simulink model "Verification_Controller_Tank2_Primitive"  (R2012b)
settings: Solver=FixedStepDiscrete  StartTime=0.0  StopTime=10.0  FixedStep=0.1  RelTol=1e-3
libraries: sldvlib x15
settings Model: Creator=Kerianne  LastModifiedBy=Kerianne
settings DataIOCC: SaveFormat=Structure
settings OptimizationCC: InlineParams=on

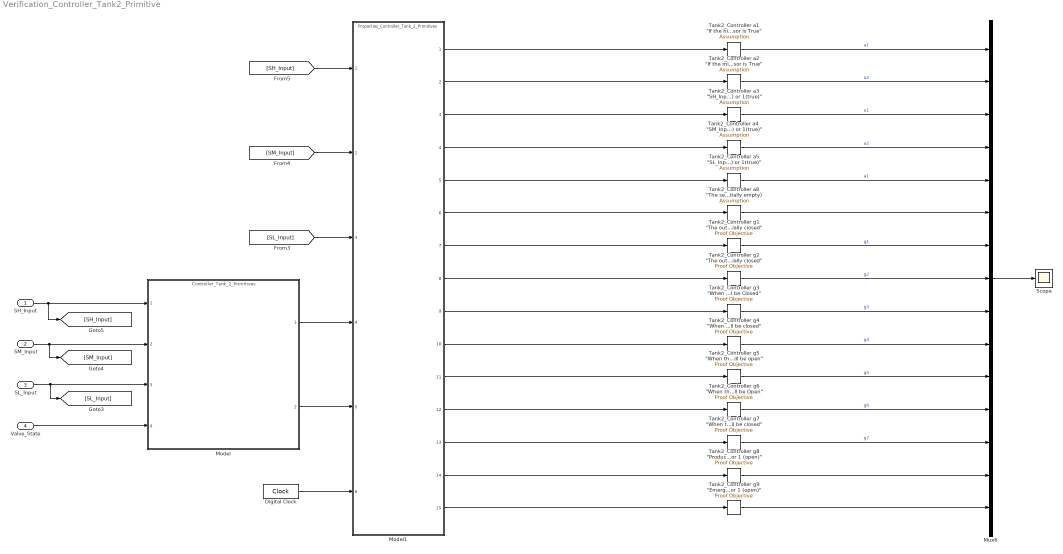
== system Verification_Controller_Tank2_Primitive ==
  SH_Input : Inport  OutDataTypeStr=double
  SM_Input : Inport  Port=2  OutDataTypeStr=double
  SL_Input : Inport  Port=3  OutDataTypeStr=double
  Valve_State : Inport  Port=4  OutDataTypeStr=double
  Digital Clock : DigitalClock  SampleTime=0.1
  Model : ModelReference  ModelNameDialog=Controller_Tank_2_Primitives  SimulationMode=Normal  ModelReferenceVersion=1.32  CopyOfModelName=Controller_Tank_2_Primitives  DefaultDataLogging=on
  Model1 : ModelReference  ModelNameDialog=Properties_Controller_Tank_2_Primitives  SimulationMode=Normal  ModelReferenceVersion=1.29  CopyOfModelName=Properties_Controller_Tank_2_Primitives  DefaultDataLogging=on
  Mux6 : Mux  Inputs=15
  Scope : Scope
      settings: ShowLegends=on
  "Tank2_Controller a1 \"If the high sensor is true, then the mid sensor is True\"" : sldvlib/Objectives and Constraints/Assumption  enabled=on  customAVTBlockType=Assumption  intervals=true  initial=off  dispValues=on  outEnabled=on
      settings: AttributesFormatString=%<intervals>
  "Tank2_Controller a2 \"If the mid sensor is true, then the low sensor is True\"" : sldvlib/Objectives and Constraints/Assumption  enabled=on  customAVTBlockType=Assumption  intervals=true  initial=off  dispValues=on  outEnabled=on
      settings: AttributesFormatString=%<intervals>
  "Tank2_Controller a3 \"SH_Input is 0 (false) or 1(true)\"" : sldvlib/Objectives and Constraints/Assumption  enabled=on  customAVTBlockType=Assumption  intervals=true  initial=off  dispValues=on  outEnabled=on
      settings: AttributesFormatString=%<intervals>
  "Tank2_Controller a4  \"SM_Input is 0 (false) or 1(true)\"" : sldvlib/Objectives and Constraints/Assumption  enabled=on  customAVTBlockType=Assumption  intervals=true  initial=off  dispValues=on  outEnabled=on
      settings: AttributesFormatString=%<intervals>
  "Tank2_Controller a5 \"SL_Input is 0 (false) or 1(true)\"" : sldvlib/Objectives and Constraints/Assumption  enabled=on  customAVTBlockType=Assumption  intervals=true  initial=off  dispValues=on  outEnabled=on
      settings: AttributesFormatString=%<intervals>
  "Tank2_Controller a8 \"The sensors are all initially false (The tanks are initially empty)" : sldvlib/Objectives and Constraints/Assumption  enabled=on  customAVTBlockType=Assumption  intervals=true  initial=off  dispValues=on  outEnabled=on
      settings: AttributesFormatString=%<intervals>
  "Tank2_Controller g1 \"The output emergency valve is initially closed\"" : sldvlib/Objectives and Constraints/Proof Objective  enabled=on  customAVTBlockType=Proof Objective  intervals=true  dispValues=on  outEnabled=on  enableStopSim=off
      settings: AttributesFormatString=%<intervals>
  "Tank2_Controller g2 \"The output production valve is initially closed\" " : sldvlib/Objectives and Constraints/Proof Objective  enabled=on  customAVTBlockType=Proof Objective  intervals=true  dispValues=on  outEnabled=on  enableStopSim=off
      settings: AttributesFormatString=%<intervals>
  "Tank2_Controller g3 \"When SL_Input is False, the valves shall be Closed\" " : sldvlib/Objectives and Constraints/Proof Objective  enabled=on  customAVTBlockType=Proof Objective  intervals=true  dispValues=on  outEnabled=on  enableStopSim=off
      settings: AttributesFormatString=%<intervals>
  "Tank2_Controller g4 \"When SM_Input is False and the SL_Input is true, the production valve shall be open and the emergency valve shall be closed\" " : sldvlib/Objectives and Constraints/Proof Objective  enabled=on  customAVTBlockType=Proof Objective  intervals=true  dispValues=on  outEnabled=on  enableStopSim=off
      settings: AttributesFormatString=%<intervals>
  "Tank2_Controller g5 \"When the SH_Input is true, both valves will be open\" " : sldvlib/Objectives and Constraints/Proof Objective  enabled=on  customAVTBlockType=Proof Objective  intervals=true  dispValues=on  outEnabled=on  enableStopSim=off
      settings: AttributesFormatString=%<intervals>
  "Tank2_Controller g6 \"When the SM_Input is True and the SH_Input is False and the emergency valve was previously open, the valves shall be Open\"" : sldvlib/Objectives and Constraints/Proof Objective  enabled=on  customAVTBlockType=Proof Objective  intervals=true  dispValues=on  outEnabled=on  enableStopSim=off
      settings: AttributesFormatString=%<intervals>
  "Tank2_Controller g7 \"When the SM_Input is True and the SH_Input is False and the emergency valve was previously closed, the production valve shall be open and the emergency valve shall be closed\"" : sldvlib/Objectives and Constraints/Proof Objective  enabled=on  customAVTBlockType=Proof Objective  intervals=true  dispValues=on  outEnabled=on  enableStopSim=off
      settings: AttributesFormatString=%<intervals>
  "Tank2_Controller g8 \"Production Valve State is 0 (closed) or 1 (open)\"" : sldvlib/Objectives and Constraints/Proof Objective  enabled=on  customAVTBlockType=Proof Objective  intervals=true  dispValues=on  outEnabled=on  enableStopSim=off
      settings: AttributesFormatString=%<intervals>
  "Tank2_Controller g9 \"Emergency Valve State is 0 (closed) or 1 (open)\"" : sldvlib/Objectives and Constraints/Proof Objective  enabled=on  customAVTBlockType=Proof Objective  intervals=true  dispValues=on  outEnabled=on  enableStopSim=off
      settings: AttributesFormatString=%<intervals>
  wires:
  SH_Input/1 -> [SH_Input], Model/1
  Model1/2 -> "Tank2_Controller a2 \"If the mid sensor is true, then the low sensor is True\""/1
  Model1/7 -> "Tank2_Controller g1 \"The output emergency valve is initially closed\""/1
  "Tank2_Controller g1 \"The output emergency valve is initially closed\""/1 -> Mux6/7  "g1"
  "Tank2_Controller a2 \"If the mid sensor is true, then the low sensor is True\""/1 -> Mux6/2  "a2"
  "Tank2_Controller a1 \"If the high sensor is true, then the mid sensor is True\""/1 -> Mux6/1  "a1"
  Model1/8 -> "Tank2_Controller g2 \"The output production valve is initially closed\" "/1
  "Tank2_Controller g2 \"The output production valve is initially closed\" "/1 -> Mux6/8  "g2"
  Model1/9 -> "Tank2_Controller g3 \"When SL_Input is False, the valves shall be Closed\" "/1
  "Tank2_Controller g3 \"When SL_Input is False, the valves shall be Closed\" "/1 -> Mux6/9  "g3"
  Model1/10 -> "Tank2_Controller g4 \"When SM_Input is False and the SL_Input is true, the production valve shall be open and the emergency valve shall be closed\" "/1
  "Tank2_Controller g4 \"When SM_Input is False and the SL_Input is true, the production valve shall be open and the emergency valve shall be closed\" "/1 -> Mux6/10  "g4"
  Model1/11 -> "Tank2_Controller g5 \"When the SH_Input is true, both valves will be open\" "/1
  "Tank2_Controller g5 \"When the SH_Input is true, both valves will be open\" "/1 -> Mux6/11  "g5"
  Model1/12 -> "Tank2_Controller g6 \"When the SM_Input is True and the SH_Input is False and the emergency valve was previously open, the valves shall be Open\""/1
  "Tank2_Controller g6 \"When the SM_Input is True and the SH_Input is False and the emergency valve was previously open, the valves shall be Open\""/1 -> Mux6/12  "g6"
  Model1/13 -> "Tank2_Controller g7 \"When the SM_Input is True and the SH_Input is False and the emergency valve was previously closed, the production valve shall be open and the emergency valve shall be closed\""/1
  "Tank2_Controller g7 \"When the SM_Input is True and the SH_Input is False and the emergency valve was previously closed, the production valve shall be open and the emergency valve shall be closed\""/1 -> Mux6/13  "g7"
  Mux6/1 -> Scope/1
  Model1/1 -> "Tank2_Controller a1 \"If the high sensor is true, then the mid sensor is True\""/1
  Model1/4 -> "Tank2_Controller a4  \"SM_Input is 0 (false) or 1(true)\""/1
  "Tank2_Controller a4  \"SM_Input is 0 (false) or 1(true)\""/1 -> Mux6/4  "a2"
  "Tank2_Controller a3 \"SH_Input is 0 (false) or 1(true)\""/1 -> Mux6/3  "a1"
  Model1/3 -> "Tank2_Controller a3 \"SH_Input is 0 (false) or 1(true)\""/1
  "Tank2_Controller a5 \"SL_Input is 0 (false) or 1(true)\""/1 -> Mux6/5  "a1"
  Model1/5 -> "Tank2_Controller a5 \"SL_Input is 0 (false) or 1(true)\""/1
  Model1/15 -> "Tank2_Controller g9 \"Emergency Valve State is 0 (closed) or 1 (open)\""/1
  "Tank2_Controller g9 \"Emergency Valve State is 0 (closed) or 1 (open)\""/1 -> Mux6/15
  "Tank2_Controller g8 \"Production Valve State is 0 (closed) or 1 (open)\""/1 -> Mux6/14
  Model1/14 -> "Tank2_Controller g8 \"Production Valve State is 0 (closed) or 1 (open)\""/1
  SM_Input/1 -> [SM_Input], Model/2
  Valve_State/1 -> Model/4
  SL_Input/1 -> [SL_Input], Model/3
  Model/2 -> Model1/5
  Model/1 -> Model1/4
  [SL_Input] -> Model1/3
  [SM_Input] -> Model1/2
  [SH_Input] -> Model1/1
  Model1/6 -> "Tank2_Controller a8 \"The sensors are all initially false (The tanks are initially empty)"/1
  "Tank2_Controller a8 \"The sensors are all initially false (The tanks are initially empty)"/1 -> Mux6/6
  Digital Clock/1 -> Model1/6
